simulink model "Airship_nonlinear_dynamics_simulink"  (R2024b)
settings: Solver=ode15s  StartTime=0.0  StopTime=1000  FixedStep=0.01  MaxStep=0.01  RelTol=1e-5  AbsTol=1e-8
InitFcn:
  | Init
values from neighbouring files (symbols this model uses):
  c = 0.465    [Init.m]    (also in Nonlinear_dynamics.m = 7; init_Skyship.m = 7)
  cf = 0.1395    [Init.m]    (also in Nonlinear_dynamics.m = 3; init_Skyship.m = 3)
  CL_alpha = 5.7    [Init.m]    (also in Nonlinear_dynamics.m; init_Skyship.m)
  D = 1.6    [Init.m]    (also in Nonlinear_dynamics.m = 14; init_Skyship.m = 14)
  delta = deg2rad(10)    [Nonlinear_dynamics.m]    (also in init_Skyship.m = -15)
  delta_e = 0    [Init.m]
  delta_r = 0    [Init.m]
  etaTDF = 1    [Init.m]    (also in Nonlinear_dynamics.m = 0.6; init_Skyship.m = 0.6)
  etaTP = 0.6    [Init.m]    (also in Nonlinear_dynamics.m; init_Skyship.m)
  fProp1 = 0    [Init.m]
  fProp2 = 0    [Init.m]
  fProp_max = 20    [Init.m]
  fTDF = 4000    [Nonlinear_dynamics.m]    (also in init_Skyship.m = 0)
  fTTP = 0    [Init.m]    (also in Nonlinear_dynamics.m = 2000; init_Skyship.m)
  FVN = [5, 5, 5]    [Init.m]    (also in Nonlinear_dynamics.m = 0; init_Skyship.m = 10)
  g = 9.81    [Init.m]    (also in Nonlinear_dynamics.m; init_Skyship.m)
  I33 = eye(3)    [Init.m]    (also in Nonlinear_dynamics.m; init_Skyship.m)
  Ixx = 1.7972    [Init.m]    (also in Nonlinear_dynamics.m = 200658; init_Skyship.m = 200658)
  Ixy = 0    [Init.m]    (also in Nonlinear_dynamics.m; init_Skyship.m)
  Ixz = 0    [Init.m]    (also in Nonlinear_dynamics.m; init_Skyship.m)
  Iyy = 4.9584    [Init.m]    (also in Nonlinear_dynamics.m = 850900; init_Skyship.m = 850900)
  Iyz = 0    [Init.m]    (also in Nonlinear_dynamics.m; init_Skyship.m)
  Izz = 7.9854    [Init.m]    (also in Nonlinear_dynamics.m = 649699; init_Skyship.m = 649699)
  k1 = keta(1)    [Init.m]    (also in Nonlinear_dynamics.m; init_Skyship.m = 0.08; ketaparameters.m = 0)
  k2 = keta(2)    [Init.m]    (also in Nonlinear_dynamics.m; init_Skyship.m = 0.89; ketaparameters.m = 0)
  k_dash = keta(3)    [Init.m]    (also in Nonlinear_dynamics.m; init_Skyship.m = 0.5; ketaparameters.m = 0)
  L = 4.7    [Init.m]    (also in Nonlinear_dynamics.m = zeros(1,4); init_Skyship.m = 52)
  m = 7.31    [Init.m]    (also in Nonlinear_dynamics.m = 5942; init_Skyship.m = 5942; velocity_tf_script.m; velocity_tf_script_v2.m)
  MAF = zeros(6,6)    [Init.m]    (also in Nonlinear_dynamics.m; init_Skyship.m)
  MVN = [0.2, 10, 5]    [Init.m]    (also in Nonlinear_dynamics.m = 0; init_Skyship.m = 0.001)
  p0 = 0    [Init.m]    (also in init_Skyship.m)
  phi0 = 0    [Init.m]    (also in init_Skyship.m)
  Prop1_alpha = 0    [Init.m]
  Prop2_alpha = 0    [Init.m]
  psi0 = 0    [Init.m]    (also in init_Skyship.m)
  q0 = 0    [Init.m]    (also in init_Skyship.m)
  r0 = 0    [Init.m]    (also in init_Skyship.m)
  rGxm = [XG-XB 0 ZG-ZB]'    [Init.m]    (also in Nonlinear_dynamics.m; init_Skyship.m)
  rho_0 = 1.225    [Init.m]    (also in Nonlinear_dynamics.m; init_Skyship.m)
  rho_he = 0.175    [Init.m]
  rTDF1 = [0 0.5 0]'    [Init.m]    (also in Nonlinear_dynamics.m = [3.5 7.87 21]'; init_Skyship.m = [3.5 7.87 21]')
  rTDF2 = [0 -0.5 0]'    [Init.m]    (also in Nonlinear_dynamics.m = [3.5 -7.87 21]'; init_Skyship.m = [3.5 -7.87 21]')
  rTTP = [0 0 0]'    [Init.m]    (also in Nonlinear_dynamics.m = [0 0 20.1]'; init_Skyship.m = [0 0 20.1]')
  Sf = 0.18135    [Init.m]    (also in Nonlinear_dynamics.m = 65; init_Skyship.m = 65)
  t_s = 0.005    [Init.m]
  theta0 = 1    [Init.m]    (also in init_Skyship.m = 0)
  u0 = 0.0    (= 0)    [Init.m]    (also in init_Skyship.m; velocity_tf_script.m = 4; velocity_tf_script_v2.m = 4)
  v0 = 0.0    (= 0)    [Init.m]    (also in init_Skyship.m)
  VB = 5.97    [Init.m]    (also in Nonlinear_dynamics.m = 5153; init_Skyship.m = 4911)
  w0 = 0.0    (= 0)    [Init.m]    (also in init_Skyship.m)
  xE0 = 0    [Init.m]    (also in init_Skyship.m)
  yE0 = 0    [Init.m]    (also in init_Skyship.m)
  zE0 = -h    (= -3.7495)    [Init.m]    (also in init_Skyship.m = -100)
undefined symbols (not defined in the file or in its folder): Sim3dSensor
libraries: slpidlib x13, simulink_extras x4, sim3dcameralib x1, sim3dlib x1, uavsim3dlib x1
(part 3 of 4)

== matlab function Airship_nonlinear_dynamics_simulink/nonlinear dynamics piecewise1/MATLAB Function6 ==
  data: phi input; g_cap output; theta input
function g_cap = fcn(phi, theta)
    g_cap = [-sin(theta), cos(theta)*sin(phi), cos(theta)*cos(phi)]';
end

== matlab function Airship_nonlinear_dynamics_simulink/nonlinear dynamics piecewise1/MATLAB Function7 ==
  data: rTDF1 input; tau_Th output; rTDF2 input; fProp1 input; fProp2 input; etaTDF input; rTTP input; fTTP input; etaTP input
function tau_Th = fcn(rTDF1, rTDF2, fProp1, fProp2, etaTDF, rTTP,  fTTP,  etaTP)
%% Airship thrust force and moments


FTDF1 = etaTDF * [fProp1 0 0 ]'; %Thrust force N
FTDF2 = etaTDF * [fProp2 0 0 ]';
FTDF = FTDF1+FTDF2;
MTDF1 = cross(rTDF1, FTDF1); %Moments N-m
MTDF2 = cross(rTDF2, FTDF2);
MTDF = MTDF1 + MTDF2;


FTTP = etaTP* [fTTP 0 0 ]';
MTTP = cross(rTTP, FTTP);

FT = FTTP + FTDF;
MT = MTTP + MTDF;
tau_Th = [FT; MT];
end

== matlab function Airship_nonlinear_dynamics_simulink/nonlinear dynamics piecewise1/V_dot out ==
  data: MAH input; V_dot output; MAF input; Mrigid input; tau_I input; tau_G input; tau_C input; tau_AS input; tau_A_dash input; tau_Th input; tau_V input
function V_dot = fcn(MAH, MAF, Mrigid,tau_I, tau_G, tau_C, tau_AS, tau_A_dash, tau_Th, tau_V)
%% Return
V_dot = zeros(6,1);
MA_rigid = (MAH+MAF);
%                                       +tau_Imp for gusts
V_dot = (MA_rigid + Mrigid) \ (tau_I + tau_G + tau_C + tau_AS + tau_A_dash + tau_Th + tau_V);
end

== matlab function Airship_nonlinear_dynamics_simulink/nonlinear dynamics piecewise1/tau_AS ==
  data: rho input; tau_AS output size=[6, 1]; g input; VB input; g_cap input; rho_he input
function tau_AS = fcn(rho, g, VB, g_cap, rho_he)
%% Aerostatic forces and moments

% first three are forces along x y z
% next three are moments along x y z 
rv = [0 0 0]'; %Since body frame is established at CV, the position ...
FAS = -(rho)*g*VB*g_cap; %Aerostatic forces N
%FAS = -((rho - rho_he) * g * VB) * g_cap;

tau_AS = [FAS; cross(rv,FAS)]; %Aerostatic forces and moments
end

== matlab function Airship_nonlinear_dynamics_simulink/Euler angle estimation2 ==
  data: phi input; EA_dot output; theta input; psi input; p input; q input; r input
function EA_dot = Euler_angle_estimation(phi, theta, psi,p, q, r)


E_dot = [1, sin(phi)* tan(theta) , cos(phi)*tan(theta);
         0, cos(phi) , -sin(phi);
         0, sin(phi)/cos(theta), cos(phi)/cos(theta)];

body_rates = [p; q; r];

EA_dot = transpose(E_dot*body_rates);

end

== matlab function Airship_nonlinear_dynamics_simulink/nonlinear dynamics piecewise1/tau_A_dash ==
  data: MA_rigid input; tau_A_dash output size=[6, 1]; omg input; V input
function tau_A_dash = fcn(MA_rigid, omg, V)
%% Aerodynamic forces and moments
% symmetric added mass axis
% Aerodynamic forces N and moments N-m

% Extract components from the symmetric added mass axis
M11 = MA_rigid(1:3, 1:3);
M12 = MA_rigid(1:3, 4:6);
M21 = MA_rigid(4:6, 1:3);
M22 = MA_rigid(4:6, 4:6);

% Calc aero forces and moments
forces_due_to_rotation = cross(omg, (M11 * V + M12 * omg));
moments_due_to_translation = cross(V, (M11 * V + M12 * omg));
moments_due_to_rotation = cross(omg, (M21 * V + M22 * omg));

% --- Pitch rate damping (natural, from hull and fins) ---
% Set this value using data for your airship (e.g. Skyship-500: -1.2e6 N·m·s/rad)
Mq = -1.2e6; % [N·m·s/rad] (example value, replace with your own if needed)
Mp = -1.2e6; % [N·m·s/rad] (example value, replace with your own if needed)

p = omg(1);

q = omg(2);  % Pitch rate (rad/s)
M_pitch_damping = Mq * q; % Negative sign already in Mq
M_yaw_damping = Mp * p; % Negative sign already in Mq

% Add pitch damping to the moment vector [L; M; N]
moments_due_to_pitch_damping = [0; M_pitch_damping; 0];
moments_due_to_yaw_damping = [M_yaw_damping;0; 0];

% Combine into aero forces and moments (sign change - to +)
tau_A_dash = [forces_due_to_rotation;
              moments_due_to_translation + moments_due_to_rotation + moments_due_to_pitch_damping+moments_due_to_yaw_damping];
end

== matlab function Airship_nonlinear_dynamics_simulink/nonlinear dynamics piecewise1/tau_C ==
  data: u input; tau_C output size=[6, 1]; v input; w input; delta_e input; delta_r input; rho input; Sf input; c input; cf input; CL_alpha input; L_hull input

function tau_C = fcn(u, v, w, delta_e, delta_r,rho, Sf, c, cf, CL_alpha, L_hull)
V_bar  = sqrt(u^2 + v^2 + w^2); % TAS m/s
S_FE   = Sf;                    % reference surface area m^2
delta_e_rad = deg2rad(delta_e);
delta_r_rad = deg2rad(delta_r);
q = 0.5 * rho * V_bar^2;
 
 %theoretical effectiveness factor tau
 theta_f = acos(2*cf/c -1);
 tau = 1- (theta_f - sin(theta_f)) /pi;
 
 %correction factor eta_d
 eta_d = 0.8; %simplified fucntion
 %3D effectiveness value
 k3D = 1.2; %example value
 %calc DeltaCL
 
 DeltaCL_elev = CL_alpha *tau * eta_d * k3D * delta_e_rad;
 DeltaCL_rud = CL_alpha *tau * eta_d * k3D * delta_r_rad;
 DeltaCD_elev = 1.7* (cf/c)^1.38 * (Sf / S_FE) * sin(delta_e_rad)^2;
 DeltaCD_rud = 1.7* (cf/c)^1.38 * (Sf / S_FE) * sin(delta_r_rad)^2; 
   %{
 %Moment calcs for each fin
 numerator = -2*sin(theta_f) - sin(2*theta_f);
 denominator = 8 * (pi - theta_f + sin(theta_f));

 ratio = numerator/denominator;

 DeltaCM1_4_elev = ratio*DeltaCL_elev;
 DeltaCM1_4_rud = ratio*DeltaCL_rud;

 %Deflection angels degrees
 theta = [90, 270, 0, 180];
  %}
 %initialize force and moment arrays
 
 Fx = zeros(1,4); %logitudinal forces
 Fy = zeros(1,4); %lateral forces
 Fz = zeros(1,4); %vertical forces
 
 L = zeros(1,4); %rolling moment
 M = zeros(1,4); %pitching moment
 N = zeros(1,4); %yawing moment
 
 %calc forces and moements for each fin
 
 for i = 1:2
 
     %calc forces
     Fx(i) = -q *Sf*DeltaCD_elev;
     Fy(i) = 0;
     Fz(i) = q*Sf*(DeltaCL_elev);
 
     L(i) = 0;
     M(i) = Fz(i)*0.5*L_hull; %assume moment arm is haf of the hull length
     N(i) = 0;
 end
 for i = 3:4
     %calc forces
     Fx(i) = -q *Sf*DeltaCD_rud;
     Fy(i) = -q *Sf*(DeltaCL_rud);
     Fz(i) = 0;
 
     L(i) = 0;
     M(i) = 0;
     N(i) = Fy(i)*0.5*L_hull; %assume moment arm is haf of the hull length
 end

 % Totals
 TotalFx = sum(Fx(:));
 TotalFy = sum(Fy(:));
 TotalFz = sum(Fz(:));

 TotalL = sum(L(:));
 TotalM = sum(M(:));
 TotalN = sum(N(:));
 tau_C = [TotalFx TotalFy TotalFz TotalL TotalM TotalN]';


end
%{
function tau_C = fcn(u, v, w, delta, rho, Sf, c, cf, CL_alpha)
% fcn computes the forces and moments exerted by the elevator.
%
% Syntax:
%   tau_C = fcn(u, v, w, delta, rho, Sf, c, cf, CL_alpha)
%
% Inputs:
%   u, v, w   - Velocities in the body axes (m/s)
%   delta     - Elevator deflection (in degrees)
%   rho       - Air density (kg/m^3)
%   Sf        - Fin (or elevator) surface area (m^2)
%   c         - Chord length of the fin (m)
%   cf        - Chord length of the flap (m)
%   CL_alpha  - Lift curve slope (per radian)
%
% Outputs:
%   tau_C     - 6x1 column vector with total force and moment components:
%               [TotalFx; TotalFy; TotalFz; TotalL; TotalM; TotalN]
%
% The function computes the force generated by the elevator using a
% simplified aerodynamic model. Later, rudder contributions can be added.
%

% -------------------------------------------------
% Constants and preliminary calculations
% -------------------------------------------------
V_bar  = sqrt(u^2 + v^2 + w^2);        % true airspeed in m/s
S_FE   = Sf;                           % reference surface area m^2
delta_rad = deg2rad(delta);            % convert deflection to radians

% Deflection angles (degrees) for all 4 fins (2 elevator and 2 rudder)
theta = [45, 135, 225, 315];

% -------------------------------------------------
% Initialize force and moment arrays
% -------------------------------------------------
% Force components (assumed to be calculated for each fin/elevator)
Fx = zeros(size(theta));  % X forces (e.g., drag)
Fy = zeros(size(theta));  % Y forces (lateral - zero in symmetric case)
Fz = zeros(size(theta));  % Z forces (lift)

% Moment components for each fin/elevator
L = zeros(size(theta));  % Rolling moment about x-axis
M = zeros(size(theta));  % Pitching moment about y-axis
N = zeros(size(theta));  % Yawing moment about z-axis

% -------------------------------------------------
% Aerodynamic force calculations
% -------------------------------------------------
% Calculate dynamic pressure
q = 0.5 * rho * V_bar^2;

% Elevator lift (simplified linear model)
% Using the relation: Lift = q * S_FE * CL_alpha * delta_rad
Lift = q * S_FE * CL_alpha * delta_rad;

% For this example, we assume that all 4 fins (or elevator surfaces)
% produce identical contributions. More nuanced models would separately
% handle the contributions from elevator vs. rudder.
%
% Here we distribute the forces and moments for each surface.
for i = 1:length(theta)
    % Forces:
    % - Fx: a small fraction (e.g., 10%) of the lift is assumed to be
    %       converted to a drag force along the x-axis.
    % - Fy: no lateral force is assumed (symmetry).
    % - Fz: the full lift is assumed to act in the vertical direction.
    Fx(i) = 0.1 * Lift;
    Fy(i) = 0;
    Fz(i) = Lift;
    
    % Moments (using chord as approximate lever arms):
    % - Rolling moment (L): assumed to be 0.5 * Lift * c
    % - Pitching moment (M): assumed to be Lift * c
    % - Yawing moment (N): assumed to be 0.5 * Lift * cf
    L(i) = 0.5 * Lift * c;
    M(i) = Lift * c;
    N(i) = 0.5 * Lift * cf;
end

% -------------------------------------------------
% Consolidate the total forces and moments
% -------------------------------------------------
TotalFx = sum(Fx(:));
TotalFy = sum(Fy(:));
TotalFz = sum(Fz(:));

TotalL  = sum(L(:));
TotalM  = sum(M(:));
TotalN  = sum(N(:));

% Output: Force and moment vector as a column vector
tau_C = [TotalFx; TotalFy; TotalFz; TotalL; TotalM; TotalN];

end
%}
%{ 
%% Control forces and moments
% Constants
 V_bar  = sqrt(v^2 + u^2 + w^2) ; %true airspeed in m/s
 S_FE = Sf; %reference surface area m^2
 delta_rad = deg2rad(delta);
 
 %theoretical effectiveness factor tau
 theta_f = acos(2*cf/c -1);
 tau = 1- (theta_f - sin(theta_f)) /pi;
 
 %correction factor eta_d
 eta_d = 0.8; %simplified fucntion
 %3D effectiveness value
 k3D = 1.2; %example value
 %calc DeltaCL
 
 DeltaCL = CL_alpha *tau * eta_d * k3D * delta_rad;
 
 DeltaCD = 1.7* (cf/c)^1.38 * (Sf / S_FE) * sin(delta_rad)^2;
 
 %Moment calcs for each fin
 numerator = -2*sin(theta_f) - sin(2*theta_f);
 denominator = 8 * (pi - theta_f + sin(theta_f));
 
 ratio = numerator/denominator;
 
 DeltaCM1_4 = ratio*DeltaCL;
 
 %Deflection angels degrees
 theta = [45, 135, 225, 315];
 
 %initialize force and moment arrays
 
 Fx = zeros(1,4);
 Fy = zeros(1,4);
 Fz = zeros(1,4);
 
 L = zeros(1,4);
 M = zeros(1,4);
 N = zeros(1,4);
 
 %calc forces and moements for each fin
 
 for i = 1:4
     %conv theta to radians
     theta_rad = deg2rad(theta(i));
 
     %calc forces
     Fx(i) = -0.5 * rho * V_bar^2 *Sf*DeltaCD;
     Fy(i) = 0.5*rho*V_bar^2*Sf*(DeltaCL *sin(theta_rad)+ DeltaCD * cos(theta_rad));
     Fz(i) = -0.5 * rho * V_bar^2 *Sf*(DeltaCL *cos(theta_rad)- DeltaCD * sin(theta_rad));
 
     L(i) = Fz(i); %Assume y_i = 1 for simplicity
     M(i) = 0.5*rho*V_bar^2*Sf*c*DeltaCM1_4;
     N(i) = Fy(i); %Assume x_i = 1 for simplicity 
 end
 % Totals
 TotalFx = sum(Fx(:));
 TotalFy = sum(Fy(:));
 TotalFz = sum(Fz(:));

 TotalL = sum(L(:));
 TotalM = sum(M(:));
 TotalN = sum(N(:));
 tau_C = [TotalFx TotalFy TotalFz TotalL TotalM TotalN]';


end
%For natural response 
%tau_C = [0 0 0 0 0 0]';
%}

== matlab function Airship_nonlinear_dynamics_simulink/nonlinear dynamics piecewise1/tau_G ==
  data: rho input; tau_G output size=[6, 1]; m input; g input; VB input; rGx input; g_cap input
function tau_G = fcn(rho, m, g, VB, rGx, g_cap)
%% Gravitational forces and moments
w = m*g;

FG = w*g_cap; % Weight component in body frame (N)
tau_G = [FG; rGx*FG];
end

== matlab function Airship_nonlinear_dynamics_simulink/nonlinear dynamics piecewise1/tau_I ==
  data: J input; tau_I output size=[6, 1]; rGx input; p input; q input; r input; V input; omg input; m input
function tau_I = fcn(J, rGx, p, q, r, V, omg,m)
%% Inertial forces (N) and moments (N-m)
omgx = [0 -omg(3) omg(2) ; omg(3) 0 -omg(1) ; -omg(2) omg(1) 0];

tau_I = [-m*omgx*V + m*omgx*rGx*omg ; -m*rGx*omgx*V - omgx*J*omg];
end

== matlab function Airship_nonlinear_dynamics_simulink/Euler angle estimation4 ==
  data: phi input; EA_dot output; theta input; psi input; p input; q input; r input
function EA_dot = Euler_angle_estimation(phi, theta, psi,p, q, r)


E_dot = [1, sin(phi)* tan(theta) , cos(phi)*tan(theta);
         0, cos(phi) , -sin(phi);
         0, sin(phi)/cos(theta), cos(phi)/cos(theta)];

body_rates = [p; q; r];

EA_dot = transpose(E_dot*body_rates);

end

== matlab function Airship_nonlinear_dynamics_simulink/Position wrt earth4 ==
  data: u input; XYZ_dot output; v input; w input; phi input; theta input; psi input
function XYZ_dot = position_wrt_Earth(u,v,w,phi,theta,psi)


R_be = [cos(theta)*cos(psi) , sin(theta)*sin(phi)*cos(psi) - cos(theta)*sin(psi), cos(phi)*cos(psi)*sin(theta)+ sin(phi)*sin(psi); ...
    cos(theta)*sin(psi), sin(phi)*sin(theta)*sin(psi) + cos(phi)*cos(psi), cos(phi)*sin(theta)*sin(psi) - sin(phi)*cos(psi); ...
    -sin(theta) , sin(phi)*cos(theta) , cos(phi)*cos(theta)];

body_velocity = [u; v; w];
XYZ_dot = transpose(R_be*body_velocity);
end

== matlab function Airship_nonlinear_dynamics_simulink/nonlinear dynamics piecewise2/MATLAB Function ==
  data: u input; V_dot output size=[6, 1]; v input; w input; p input; q input; r input; phi input; theta input; psi input; Z input; MAF input; m input; I33 input; rGxm input; Ixx input; Iyy input; Izz input; Ixy input; Ixz input; Iyz input; g input; L input; D input; k1 input; k2 input; k_dash input; VB input; delta input; rTDF1 input; rTDF2 input; fTDF input; etaTDF input; rTTP input; fTTP input; etaTP input
function V_dot = fcn(u, v, w, p, q, r, phi, theta, psi, Z, MAF, m, I33, rGxm, Ixx, Iyy, Izz, Ixy, Ixz, Iyz, g, L, D, k1, k2, k_dash, VB, delta, rTDF1, rTDF2, fTDF, etaTDF, rTTP,  fTTP,  etaTP)
rGx = [0 -rGxm(3) rGxm(2) ; rGxm(3) 0 -rGxm(1) ; -rGxm(2) rGxm(1) 0];
J = [ Ixx, Ixy, Ixz ; Ixy, Iyy, Iyz ; Ixz, Iyz, Izz];
Mrigid = [m*I33, -m*rGx; m*rGx,  J];
g_cap = [-sin(theta), cos(theta)*sin(phi), cos(theta)*cos(phi)]';
V = [u v w]';
omg = [p q r]';
altitude = -Z;
rho_0 = 1.225; %Density at sea level in kg/m3
H = 8400; %Scale height in meters;
%alitude range
%altitude = -airship(12); %linspace(0,12000, 500); %Altitude from 0 to 12000 m
density = rho_0 *exp(-altitude / H );
rho = density;

%% Estimation of added mass matrix
% MAH - added mass of airship hull
B = VB*rho*g; %Bouyancy force
m_dash = B/g;
%I_dash = sum(m_dash * (L.^2 + D^2) / 20); 
I_dash = (m_dash * (L.^2 + D^2) / 20); 
mH11 = k1*m_dash;
mH22 = k2*m_dash;
mH33 = mH22;
mH44 = 0;
mH55 = k_dash*I_dash;
mH66 = mH55;
mH = [mH11, mH22, mH33, mH44, mH55, mH66];
MAH = diag(mH); %6x6 diagonal matrix

MA_rigid = (MAH+MAF);

%% Inertial forces (N) and moments (N-m)
omgx = [0 -omg(3) omg(2) ; omg(3) 0 -omg(1) ; -omg(2) omg(1) 0];
tau_I = [-m*omgx*V + m*omgx*rGx*omg ; -m*rGx*omgx*V - omgx*J*omg];

%% Gravitational forces and moments
w = m*g;
B = VB*rho*g;
FG = w*g_cap; % Weight component in body frame (N)
tau_G = [FG; rGx*FG];

%% Control forces and moments
% Constants

 V_bar  = sqrt(v^2 + u^2 + w^2) ; %true airspeed in m/s
 Sf = 65; % Surface area of the fin m^2
 c= 7 ; % Chord length of the fin
 cf = 3; %Flap chord
 
 S_FE = 65; %reference surface area m^2
 %
 delta_rad = deg2rad(delta);
 %lift curve slope
 CL_alpha = 5.7; %Change as needed
 
 %theoretical effectiveness factor tau
 theta_f = acos(2*cf/c -1);
 tau = 1- (theta_f - sin(theta_f)) /pi;
 
 %correction factor eta_d
 eta_d = 0.8; %simplified fucntion
 %3D effectiveness value
 k3D = 1.2; %example value
 %calc DeltaCL
 
 DeltaCL = CL_alpha *tau * eta_d * k3D * delta_rad;
 
 DeltaCD = 1.7* (cf/c)^1.38 * (Sf / S_FE) * sin(delta_rad)^2;
 
 %Moment calcs for each fin
 numerator = -2*sin(theta_f) - sin(2*theta_f);
 denominator = 8 * (pi - theta_f + sin(theta_f));
 
 ratio = numerator/denominator;
 
 DeltaCM1_4 = ratio*DeltaCL;
 
 %Deflection anges degrees
 theta = [45, 135, 225, 315];
 
 %initialize force and moment arrays
 
 Fx = zeros(1,4);
 Fy = zeros(1,4);
 Fz = zeros(1,4);
 
 L = zeros(1,4);
 M = zeros(1,4);
 N = zeros(1,4);
 
 %calc forces and moements for each fin
 
 for i = 1:4
     %conv theta to radians
     theta_rad = deg2rad(theta(i));
 
     %calc forces
     Fx(i) = -0.5 * rho * V_bar^2 *Sf*DeltaCD;
     Fy(i) = 0.5*rho*V_bar^2*Sf*(DeltaCL *sin(theta_rad)+ DeltaCD * cos(theta_rad));
     Fz(i) = -0.5 * rho * V_bar^2 *Sf*(DeltaCL *cos(theta_rad)- DeltaCD * sin(theta_rad));
 
     L(i) = Fz(i); %Assume y_i = 1 for simplicity
     M(i) = 0.5*rho*V_bar^2*Sf*c*DeltaCM1_4;
     N(i) = Fy(i); %Assume x_i = 1 for simplicity 
 end
 % Totals
 TotalFx = sum(Fx(:));
 TotalFy = sum(Fy(:));
 TotalFz = sum(Fz(:));

 TotalL = sum(L(:));
 TotalM = sum(M(:));
 TotalN = sum(N(:));
 tau_C = [TotalFx TotalFy TotalFz TotalL TotalM TotalN]';
%For natural response 
%tau_C = [0 0 0 0 0 0]';

%% Aerostatic forces and moments

% first three are forces along x y z
% next three are moments along x y z 
rv = [0 0 0]'; %Since body frame is established at CV, the position ...
FAS = -rho*g*VB*g_cap; %Aerostatic forces N
tau_AS = [FAS; cross(rv,FAS)]; %Aerostatic forces and moments

%% Aerodynamic forces and moments
% symmetric added mass axis
% Aerodynamic forces N and moments N-m

%extract components from the syymetric added mass axis
M11 = MA_rigid(1:3, 1:3);
M12 = MA_rigid(1:3, 4:6);
M21 = MA_rigid(4:6, 1:3);
M22 = MA_rigid(4:6, 4:6);

% Calc aero forces and moments

forces_due_to_rotation = cross(omg, (M11 * V + M12 *omg));
moments_due_to_translation = cross(V, (M11*V+M12*omg));
moments_due_to_rotation = cross (omg, (M21*V + M22*omg));

tau_A_dash = zeros(6,1);
%combine into aero forces and moments (sign change - to +)
tau_A_dash = [forces_due_to_rotation; moments_due_to_translation+moments_due_to_rotation];

%% Airship thrust force and moments


FTDF1 = etaTDF * [fTDF 0 0 ]'; %Thrust force N
FTDF2 = etaTDF * [fTDF 0 0 ]';
FTDF = FTDF1+FTDF2;
MTDF1 = cross(rTDF1, FTDF1); %Moments N-m
MTDF2 = cross(rTDF2, FTDF2);
MTDF = MTDF1 + MTDF2;


FTTP = etaTP* [fTTP 0 0 ]';
MTTP = cross(rTTP, FTTP);

FT = FTTP + FTDF;
MT = MTTP + MTDF;
tau_Th = [FT; MT];

%% Viscous forces
FVN = 0; %Viscous force
MVN = 0; %Viscous Moment

if v == 0 && w == 0
    FV = [0 0 0]';
    MV = [0 0 0]';
else
    FV = FVN*[0 (-v/sqrt(v^2 + w^2)) (-w/sqrt(v^2 +w^2)) ]';
    MV = MVN*[0 (w/sqrt(v^2 + w^2)) (-v/sqrt(v^2 +w^2)) ]';
end
tau_V = [FV; MV];

%tau_V = [0 0 0 0 0 0]'; %if slow speed


%% Return
V_dot = zeros(6,1);
MA_rigid = (MAH+MAF);


%                                       +tau_Imp for gusts
V_dot = (MA_rigid + Mrigid) \ (tau_I + tau_G + tau_C + tau_AS + tau_A_dash + tau_Th + tau_V);

== matlab function Airship_nonlinear_dynamics_simulink/nonlinear dynamics piecewise/tau_I ==
  data: J input; tau_I output size=[6, 1]; rGx input; p input; q input; r input; V input; omg input
function tau_I = fcn(J, rGx, p, q, r, V, omg)
%% Inertial forces (N) and moments (N-m)
omgx = [0 -omg(3) omg(2) ; omg(3) 0 -omg(1) ; -omg(2) omg(1) 0];

tau_I = [-m*omgx*V + m*omgx*rGx*omg ; -m*rGx*omgx*V - omgx*J*omg];

== matlab function Airship_nonlinear_dynamics_simulink/Airship_model/Euler angle estimation5 ==
  data: phi input; EA_dot output; theta input; psi input; p input; q input; r input
function EA_dot = Euler_angle_estimation(phi, theta, psi,p, q, r)


E_dot = [1, sin(phi)* tan(theta) , cos(phi)*tan(theta);
         0, cos(phi) , -sin(phi);
         0, sin(phi)/cos(theta), cos(phi)/cos(theta)];

body_rates = [p; q; r];

EA_dot = transpose(E_dot*body_rates);

end

== matlab function Airship_nonlinear_dynamics_simulink/Airship_model/Position wrt earth5 ==
  data: u input; XYZ_dot output; v input; w input; phi input; theta input; psi input
function XYZ_dot = position_wrt_Earth(u,v,w,phi,theta,psi)


R_be = [cos(theta)*cos(psi) , sin(theta)*sin(phi)*cos(psi) - cos(theta)*sin(psi), cos(phi)*cos(psi)*sin(theta)+ sin(phi)*sin(psi); ...
    cos(theta)*sin(psi), sin(phi)*sin(theta)*sin(psi) + cos(phi)*cos(psi), cos(phi)*sin(theta)*sin(psi) - sin(phi)*cos(psi); ...
    -sin(theta) , sin(phi)*cos(theta) , cos(phi)*cos(theta)];

body_velocity = [u; v; w];
XYZ_dot = transpose(R_be*body_velocity);
end

== matlab function Airship_nonlinear_dynamics_simulink/Airship_model/nonlinear dynamics piecewise3/MAH ==
  data: MAH output; g input; L input; D input; k1 input; k2 input; k_dash input; VB input; rho input
function MAH = fcn(g, L, D, k1, k2, k_dash, VB, rho)
%% Estimation of added mass matrix
% MAH - added mass of airship hull
B = VB*rho*g; %Bouyancy force
m_dash = B/g;
%I_dash = sum(m_dash * (L.^2 + D^2) / 20); 
I_dash = (m_dash * (L.^2 + D^2) / 20); 

mH11 = k1*m_dash;
mH22 = k2*m_dash;
mH33 = mH22;
mH44 = 0;
mH55 = k_dash*I_dash;
mH66 = mH55;
mH = [mH11, mH22, mH33, mH44, mH55, mH66];

MAH = diag(mH); %6x6 diagonal matrix
end

== matlab function Airship_nonlinear_dynamics_simulink/Airship_model/nonlinear dynamics piecewise3/MATLAB Function10 ==
  data: u input; V output; v input; w input
function V = fcn(u, v, w)
V = [u v w]';
end

== matlab function Airship_nonlinear_dynamics_simulink/Airship_model/nonlinear dynamics piecewise3/MATLAB Function11 ==
  data: V input; r input; q input; tau_V output size=[6,1]; MVN input; FVN input
 function tau_V = fcn(V, r,q, MVN, FVN)
 u= V(1); 
 v = V(2);
 w= V(3);

 if v == 0 && w == 0
     FV = [0 0 0]';
     MV = [0 0 0]';
 else
     FV = FVN.*[-u (-v) (-w) ]';
     %FV = FVN*[0 (-v/sqrt(v^2 + w^2)) (-w/sqrt(v^2 +w^2)) ]';
     %MV = MVN*[0 (w/sqrt(v^2 + w^2)) (-v/sqrt(v^2 +w^2)) ]';
    MV = MVN.*[0 (w) (-v) ]'; %make first element function of p if roll oscilations persists

 end
 MV(3) = MV(3) - MVN(3) * r; 
 MV(2) = MV(2) - MVN(2) * q;
 tau_V = [FV; MV];
 %tau_V = [0 0 0 0 0 0]'; %if slow speed
 
 end

== matlab function Airship_nonlinear_dynamics_simulink/Airship_model/nonlinear dynamics piecewise3/MATLAB Function14 ==
  data: altitude input; rho output; rho_0 input
function rho = fcn(altitude, rho_0)
    % Constants
    T0 = 288.15;     % K
    L = 0.0065;      % K/m
    g = 9.80665;     % m/s^2
    R = 287.05;      % J/kg.K
%altitude = max(0, altitude);  % keep ≥ 0, but not forcefully clipped
    term = 1 - (L * altitude) / T0;
%rho= rho_0;
    if term <= 0
        rho = 0;
    else
       rho = rho_0 * term^(g / (R * L));
    end
end

== matlab function Airship_nonlinear_dynamics_simulink/Airship_model/nonlinear dynamics piecewise3/MATLAB Function15 ==
  data: p input; omg output; q input; r input
function omg = fcn(p, q, r)
omg = [p q r]';
end

== matlab function Airship_nonlinear_dynamics_simulink/Airship_model/nonlinear dynamics piecewise3/MATLAB Function2 ==
  data: rGxm input; rGx output
function rGx = fcn(rGxm)
rGx = [0 -rGxm(3) rGxm(2) ; rGxm(3) 0 -rGxm(1) ; -rGxm(2) rGxm(1) 0];

end

== matlab function Airship_nonlinear_dynamics_simulink/Airship_model/nonlinear dynamics piecewise3/MATLAB Function3 ==
  data: Ixx input; J output; Iyy input; Izz input; Ixy input; Ixz input; Iyz input
function J = fcn(Ixx, Iyy, Izz, Ixy, Ixz, Iyz)
J = [ Ixx, Ixy, Ixz ; Ixy, Iyy, Iyz ; Ixz, Iyz, Izz];
end

== matlab function Airship_nonlinear_dynamics_simulink/Airship_model/nonlinear dynamics piecewise3/MATLAB Function4 ==
  data: m input; Mrigid output; I33 input; rGx input; J input
function Mrigid = fcn(m, I33, rGx, J)
Mrigid = [m*I33, -m*rGx; m*rGx,  J];

end

== matlab function Airship_nonlinear_dynamics_simulink/Airship_model/nonlinear dynamics piecewise3/MATLAB Function6 ==
  data: phi input; g_cap output; theta input
function g_cap = fcn(phi, theta)
    g_cap = [-sin(theta), cos(theta)*sin(phi), cos(theta)*cos(phi)]';
end

== matlab function Airship_nonlinear_dynamics_simulink/Airship_model/nonlinear dynamics piecewise3/MATLAB Function7 ==
  data: rTDF1 input; tau_Th output; rTDF2 input; fProp1 input; fProp2 input; etaTDF input; Prop1_alpha input; Prop2_alpha input
function tau_Th = fcn(rTDF1, rTDF2, fProp1, fProp2, etaTDF, Prop1_alpha, Prop2_alpha)
%% Airship thrust force and moments


FTDF1 = etaTDF * [fProp1*cos(Prop1_alpha) 0 -fProp1*sin(Prop1_alpha)]'; %Thrust force N
FTDF2 = etaTDF * [fProp2*cos(Prop2_alpha) 0 -fProp2*sin(Prop2_alpha)]';
FTDF = FTDF1+FTDF2;
MTDF1 = cross(rTDF1, FTDF1); %Moments N-m
MTDF2 = cross(rTDF2, FTDF2);
MTDF = MTDF1 + MTDF2;

tau_Th = [FTDF; MTDF];
end

== matlab function Airship_nonlinear_dynamics_simulink/Airship_model/nonlinear dynamics piecewise3/V_dot out ==
  data: MAH input; V_dot output; MAF input; Mrigid input; tau_I input; tau_G input; tau_C input; tau_AS input; tau_A_dash input; tau_Th input; tau_V input
function V_dot = fcn(MAH, MAF, Mrigid,tau_I, tau_G, tau_C, tau_AS, tau_A_dash, tau_Th, tau_V)
%% Return
V_dot = zeros(6,1);
MA_rigid = (MAH+MAF);
%                                       +tau_Imp for gusts
V_dot = (MA_rigid + Mrigid) \ (tau_I + tau_G + tau_C + tau_AS + tau_A_dash + tau_Th + tau_V);
end

== matlab function Airship_nonlinear_dynamics_simulink/Position wrt earth2 ==
  data: u input; XYZ_dot output; v input; w input; phi input; theta input; psi input
function XYZ_dot = position_wrt_Earth(u,v,w,phi,theta,psi)


R_be = [cos(theta)*cos(psi) , sin(theta)*sin(phi)*cos(psi) - cos(theta)*sin(psi), cos(phi)*cos(psi)*sin(theta)+ sin(phi)*sin(psi); ...
    cos(theta)*sin(psi), sin(phi)*sin(theta)*sin(psi) + cos(phi)*cos(psi), cos(phi)*sin(theta)*sin(psi) - sin(phi)*cos(psi); ...
    -sin(theta) , sin(phi)*cos(theta) , cos(phi)*cos(theta)];

body_velocity = [u; v; w];
XYZ_dot = transpose(R_be*body_velocity);
end

== matlab function Airship_nonlinear_dynamics_simulink/Airship_model/nonlinear dynamics piecewise3/tau_AS ==
  data: rho input; tau_AS output size=[6, 1]; g input; VB input; g_cap input; rho_he input
function tau_AS = fcn(rho, g, VB, g_cap, rho_he)
%% Aerostatic forces and moments

% first three are forces along x y z
% next three are moments along x y z 
rv = [0 0 0]'; %Since body frame is established at CV, the position vector is 0
FAS = -(rho)*g*VB*g_cap; %Aerostatic forces N
%FAS = -((rho - rho_he) * g * VB) * g_cap;

tau_AS = [FAS; cross(rv,FAS)]; %Aerostatic forces and moments
end

== matlab function Airship_nonlinear_dynamics_simulink/Airship_model/nonlinear dynamics piecewise3/tau_A_dash ==
  data: MA_rigid input; tau_A_dash output size=[6, 1]; omg input; V input
function tau_A_dash = fcn(MA_rigid, omg, V)
%% Aerodynamic forces and moments
% symmetric added mass axis
% Aerodynamic forces N and moments N-m

% Extract components from the symmetric added mass axis
M11 = MA_rigid(1:3, 1:3);
M12 = MA_rigid(1:3, 4:6);
M21 = MA_rigid(4:6, 1:3);
M22 = MA_rigid(4:6, 4:6);

% Calc aero forces and moments
forces_due_to_rotation = cross(omg, (M11 * V + M12 * omg));
moments_due_to_translation = cross(V, (M11 * V + M12 * omg));
moments_due_to_rotation = cross(omg, (M21 * V + M22 * omg));

% --- Pitch rate damping (natural, from hull and fins) ---
% Set this value using data for your airship (e.g. Skyship-500: -1.2e6 N·m·s/rad)
Mq = -1.2e6; % [N·m·s/rad] (example value, replace with your own if needed)
Mp = -1.2e6; % [N·m·s/rad] (example value, replace with your own if needed)

p = omg(1);

q = omg(2);  % Pitch rate (rad/s)
M_pitch_damping = Mq * q; % Negative sign already in Mq
M_yaw_damping = Mp * p; % Negative sign already in Mq

% Add pitch damping to the moment vector [L; M; N]
moments_due_to_pitch_damping = [0; M_pitch_damping; 0];
moments_due_to_yaw_damping = [M_yaw_damping;0; 0];

% Combine into aero forces and moments (sign change - to +)
tau_A_dash = [forces_due_to_rotation;
              moments_due_to_translation + moments_due_to_rotation + moments_due_to_pitch_damping+moments_due_to_yaw_damping];
end

== matlab function Airship_nonlinear_dynamics_simulink/Airship_model/nonlinear dynamics piecewise3/tau_C ==
  data: u input; tau_C output size=[6, 1]; v input; w input; delta_e input; delta_r input; rho input; Sf input; c input; cf input; CL_alpha input; L_hull input

function tau_C = fcn(u, v, w, delta_e, delta_r,rho, Sf, c, cf, CL_alpha, L_hull)
V_bar  = sqrt(u^2 + v^2 + w^2); % TAS m/s
S_FE   = Sf;                    % reference surface area m^2
delta_e_rad = deg2rad(delta_e);
delta_r_rad = deg2rad(delta_r);
q = 0.5 * rho * V_bar^2;
 
 %theoretical effectiveness factor tau
 theta_f = acos(2*cf/c -1);
 tau = 1- (theta_f - sin(theta_f)) /pi;
 
 %correction factor eta_d
 eta_d = 0.8; %simplified fucntion
 %3D effectiveness value
 k3D = 1.2; %example value
 %calc DeltaCL
 
 DeltaCL_elev = CL_alpha *tau * eta_d * k3D * delta_e_rad;
 DeltaCL_rud = CL_alpha *tau * eta_d * k3D * delta_r_rad;
 DeltaCD_elev = 1.7* (cf/c)^1.38 * (Sf / S_FE) * sin(delta_e_rad)^2;
 DeltaCD_rud = 1.7* (cf/c)^1.38 * (Sf / S_FE) * sin(delta_r_rad)^2; 
   %{
 %Moment calcs for each fin
 numerator = -2*sin(theta_f) - sin(2*theta_f);
 denominator = 8 * (pi - theta_f + sin(theta_f));

 ratio = numerator/denominator;

 DeltaCM1_4_elev = ratio*DeltaCL_elev;
 DeltaCM1_4_rud = ratio*DeltaCL_rud;

 %Deflection angels degrees
 theta = [90, 270, 0, 180];
  %}
 %initialize force and moment arrays
 
 Fx = zeros(1,4); %logitudinal forces
 Fy = zeros(1,4); %lateral forces
 Fz = zeros(1,4); %vertical forces
 
 L = zeros(1,4); %rolling moment
 M = zeros(1,4); %pitching moment
 N = zeros(1,4); %yawing moment
 
 %calc forces and moements for each fin
 
 for i = 1:2
 
     %calc forces
     Fx(i) = -q *Sf*DeltaCD_elev;
     Fy(i) = 0;
     Fz(i) = -q*Sf*(DeltaCL_elev);
 
     L(i) = 0;
     M(i) = Fz(i)*0.5*L_hull; %assume moment arm is haf of the hull length
     N(i) = 0;
 end
 for i = 3:4
     %calc forces
     Fx(i) = -q *Sf*DeltaCD_rud;
     Fy(i) = q *Sf*(DeltaCL_rud);
     Fz(i) = 0;
 
     L(i) = 0;
     M(i) = 0;
     N(i) = Fy(i)*0.5*L_hull; %assume moment arm is haf of the hull length
 end

 % Totals
 TotalFx = sum(Fx(:));
 TotalFy = sum(Fy(:));
 TotalFz = sum(Fz(:));

 TotalL = sum(L(:));
 TotalM = sum(M(:));
 TotalN = sum(N(:));
 tau_C = [TotalFx TotalFy TotalFz TotalL TotalM TotalN]';


end
%{
function tau_C = fcn(u, v, w, delta, rho, Sf, c, cf, CL_alpha)
% fcn computes the forces and moments exerted by the elevator.
%
% Syntax:
%   tau_C = fcn(u, v, w, delta, rho, Sf, c, cf, CL_alpha)
%
% Inputs:
%   u, v, w   - Velocities in the body axes (m/s)
%   delta     - Elevator deflection (in degrees)
%   rho       - Air density (kg/m^3)
%   Sf        - Fin (or elevator) surface area (m^2)
%   c         - Chord length of the fin (m)
%   cf        - Chord length of the flap (m)
%   CL_alpha  - Lift curve slope (per radian)
%
% Outputs:
%   tau_C     - 6x1 column vector with total force and moment components:
%               [TotalFx; TotalFy; TotalFz; TotalL; TotalM; TotalN]
%
% The function computes the force generated by the elevator using a
% simplified aerodynamic model. Later, rudder contributions can be added.
%

% -------------------------------------------------
% Constants and preliminary calculations
% -------------------------------------------------
V_bar  = sqrt(u^2 + v^2 + w^2);        % true airspeed in m/s
S_FE   = Sf;                           % reference surface area m^2
delta_rad = deg2rad(delta);            % convert deflection to radians

% Deflection angles (degrees) for all 4 fins (2 elevator and 2 rudder)
theta = [45, 135, 225, 315];

% -------------------------------------------------
% Initialize force and moment arrays
% -------------------------------------------------
% Force components (assumed to be calculated for each fin/elevator)
Fx = zeros(size(theta));  % X forces (e.g., drag)
Fy = zeros(size(theta));  % Y forces (lateral - zero in symmetric case)
Fz = zeros(size(theta));  % Z forces (lift)

% Moment components for each fin/elevator
L = zeros(size(theta));  % Rolling moment about x-axis
M = zeros(size(theta));  % Pitching moment about y-axis
N = zeros(size(theta));  % Yawing moment about z-axis

% -------------------------------------------------
% Aerodynamic force calculations
% -------------------------------------------------
% Calculate dynamic pressure
q = 0.5 * rho * V_bar^2;

% Elevator lift (simplified linear model)
% Using the relation: Lift = q * S_FE * CL_alpha * delta_rad
Lift = q * S_FE * CL_alpha * delta_rad;

% For this example, we assume that all 4 fins (or elevator surfaces)
% produce identical contributions. More nuanced models would separately
% handle the contributions from elevator vs. rudder.
%
% Here we distribute the forces and moments for each surface.
for i = 1:length(theta)
    % Forces:
    % - Fx: a small fraction (e.g., 10%) of the lift is assumed to be
    %       converted to a drag force along the x-axis.
    % - Fy: no lateral force is assumed (symmetry).
    % - Fz: the full lift is assumed to act in the vertical direction.
    Fx(i) = 0.1 * Lift;
    Fy(i) = 0;
    Fz(i) = Lift;
    
    % Moments (using chord as approximate lever arms):
    % - Rolling moment (L): assumed to be 0.5 * Lift * c
    % - Pitching moment (M): assumed to be Lift * c
    % - Yawing moment (N): assumed to be 0.5 * Lift * cf
    L(i) = 0.5 * Lift * c;
    M(i) = Lift * c;
    N(i) = 0.5 * Lift * cf;
end

% -------------------------------------------------
% Consolidate the total forces and moments
% -------------------------------------------------
TotalFx = sum(Fx(:));
TotalFy = sum(Fy(:));
TotalFz = sum(Fz(:));

TotalL  = sum(L(:));
TotalM  = sum(M(:));
TotalN  = sum(N(:));

% Output: Force and moment vector as a column vector
tau_C = [TotalFx; TotalFy; TotalFz; TotalL; TotalM; TotalN];

end
%}
%{ 
%% Control forces and moments
% Constants
 V_bar  = sqrt(v^2 + u^2 + w^2) ; %true airspeed in m/s
 S_FE = Sf; %reference surface area m^2
 delta_rad = deg2rad(delta);
 
 %theoretical effectiveness factor tau
 theta_f = acos(2*cf/c -1);
 tau = 1- (theta_f - sin(theta_f)) /pi;
 
 %correction factor eta_d
 eta_d = 0.8; %simplified fucntion
 %3D effectiveness value
 k3D = 1.2; %example value
 %calc DeltaCL
 
 DeltaCL = CL_alpha *tau * eta_d * k3D * delta_rad;
 
 DeltaCD = 1.7* (cf/c)^1.38 * (Sf / S_FE) * sin(delta_rad)^2;
 
 %Moment calcs for each fin
 numerator = -2*sin(theta_f) - sin(2*theta_f);
 denominator = 8 * (pi - theta_f + sin(theta_f));
 
 ratio = numerator/denominator;
 
 DeltaCM1_4 = ratio*DeltaCL;
 
 %Deflection angels degrees
 theta = [45, 135, 225, 315];
 
 %initialize force and moment arrays
 
 Fx = zeros(1,4);
 Fy = zeros(1,4);
 Fz = zeros(1,4);
 
 L = zeros(1,4);
 M = zeros(1,4);
 N = zeros(1,4);
 
 %calc forces and moements for each fin
 
 for i = 1:4
     %conv theta to radians
     theta_rad = deg2rad(theta(i));
 
     %calc forces
     Fx(i) = -0.5 * rho * V_bar^2 *Sf*DeltaCD;
     Fy(i) = 0.5*rho*V_bar^2*Sf*(DeltaCL *sin(theta_rad)+ DeltaCD * cos(theta_rad));
     Fz(i) = -0.5 * rho * V_bar^2 *Sf*(DeltaCL *cos(theta_rad)- DeltaCD * sin(theta_rad));
 
     L(i) = Fz(i); %Assume y_i = 1 for simplicity
     M(i) = 0.5*rho*V_bar^2*Sf*c*DeltaCM1_4;
     N(i) = Fy(i); %Assume x_i = 1 for simplicity 
 end
 % Totals
 TotalFx = sum(Fx(:));
 TotalFy = sum(Fy(:));
 TotalFz = sum(Fz(:));

 TotalL = sum(L(:));
 TotalM = sum(M(:));
 TotalN = sum(N(:));
 tau_C = [TotalFx TotalFy TotalFz TotalL TotalM TotalN]';


end
%For natural response 
%tau_C = [0 0 0 0 0 0]';
%}

== matlab function Airship_nonlinear_dynamics_simulink/Airship_model/nonlinear dynamics piecewise3/tau_G ==
  data: rho input; tau_G output size=[6, 1]; m input; g input; VB input; rGx input; g_cap input
function tau_G = fcn(rho, m, g, VB, rGx, g_cap)
%% Gravitational forces and moments
w = m*g;

FG = w*g_cap; % Weight component in body frame (N)
tau_G = [FG; rGx*FG];
end

== matlab function Airship_nonlinear_dynamics_simulink/Airship_model/nonlinear dynamics piecewise3/tau_I ==
  data: J input; tau_I output size=[6, 1]; rGx input; p input; q input; r input; V input; omg input; m input
function tau_I = fcn(J, rGx, p, q, r, V, omg,m)
%% Inertial forces (N) and moments (N-m)
omgx = [0 -omg(3) omg(2) ; omg(3) 0 -omg(1) ; -omg(2) omg(1) 0];

tau_I = [-m*omgx*V + m*omgx*rGx*omg ; -m*rGx*omgx*V - omgx*J*omg];
end

== matlab function Airship_nonlinear_dynamics_simulink/MATLAB Function ==
  data: t input; y output
function y = fcn(t)
if t < 5 
    y = 5; 
elseif t < 15 
    y = 0; 
elseif t < 20
    y = -5; 
elseif t < 30
    y = 0; 
elseif t <35 
    y = -5; 
elseif t <45 
    y = 0; 
elseif t <50 
    y = 5; 
elseif t<60
    y=-0;

else 
    y = 0;
end 
end

== matlab function Airship_nonlinear_dynamics_simulink/Airship_model1/Euler angle estimation5 ==
  data: phi input; EA_dot output; theta input; psi input; p input; q input; r input
function EA_dot = Euler_angle_estimation(phi, theta, psi,p, q, r)


E_dot = [1, sin(phi)* tan(theta) , cos(phi)*tan(theta);
         0, cos(phi) , -sin(phi);
         0, sin(phi)/cos(theta), cos(phi)/cos(theta)];

body_rates = [p; q; r];

EA_dot = transpose(E_dot*body_rates);

end

== matlab function Airship_nonlinear_dynamics_simulink/Airship_model1/Position wrt earth5 ==
  data: u input; XYZ_dot output; v input; w input; phi input; theta input; psi input
function XYZ_dot = position_wrt_Earth(u,v,w,phi,theta,psi)


R_be = [cos(theta)*cos(psi) , sin(theta)*sin(phi)*cos(psi) - cos(theta)*sin(psi), cos(phi)*cos(psi)*sin(theta)+ sin(phi)*sin(psi); ...
    cos(theta)*sin(psi), sin(phi)*sin(theta)*sin(psi) + cos(phi)*cos(psi), cos(phi)*sin(theta)*sin(psi) - sin(phi)*cos(psi); ...
    -sin(theta) , sin(phi)*cos(theta) , cos(phi)*cos(theta)];

body_velocity = [u; v; w];
XYZ_dot = transpose(R_be*body_velocity);
end

== matlab function Airship_nonlinear_dynamics_simulink/Airship_model1/nonlinear dynamics piecewise3/MAH ==
  data: MAH output; g input; L input; D input; k1 input; k2 input; k_dash input; VB input; rho input
function MAH = fcn(g, L, D, k1, k2, k_dash, VB, rho)
%% Estimation of added mass matrix
% MAH - added mass of airship hull
B = VB*rho*g; %Bouyancy force
m_dash = B/g;
%I_dash = sum(m_dash * (L.^2 + D^2) / 20); 
I_dash = (m_dash * (L.^2 + D^2) / 20); 

mH11 = k1*m_dash;
mH22 = k2*m_dash;
mH33 = mH22;
mH44 = 0;
mH55 = k_dash*I_dash;
mH66 = mH55;
mH = [mH11, mH22, mH33, mH44, mH55, mH66];

MAH = diag(mH); %6x6 diagonal matrix
end

== matlab function Airship_nonlinear_dynamics_simulink/Euler angle estimation1 ==
  data: phi input; EA_dot output; theta input; psi input; p input; q input; r input
function EA_dot = Euler_angle_estimation(phi, theta, psi,p, q, r)


E_dot = [1, sin(phi)* tan(theta) , cos(phi)*tan(theta);
         0, cos(phi) , -sin(phi);
         0, sin(phi)/cos(theta), cos(phi)/cos(theta)];

body_rates = [p; q; r];

EA_dot = transpose(E_dot*body_rates);

end

== matlab function Airship_nonlinear_dynamics_simulink/Airship_model1/nonlinear dynamics piecewise3/MATLAB Function10 ==
  data: u input; V output; v input; w input
function V = fcn(u, v, w)
V = [u v w]';
end

== matlab function Airship_nonlinear_dynamics_simulink/Airship_model1/nonlinear dynamics piecewise3/MATLAB Function11 ==
  data: V input; r input; tau_V output size=[6,1]; MVN input; FVN input
 function tau_V = fcn(V, r, MVN, FVN)
 u= V(1); 
 v = V(2);
 w= V(3);

 if v == 0 && w == 0
     FV = [0 0 0]';
     MV = [0 0 0]';
 else
     FV = FVN.*[-u (-v) (-w) ]';
     %FV = FVN*[0 (-v/sqrt(v^2 + w^2)) (-w/sqrt(v^2 +w^2)) ]';
     %MV = MVN*[0 (w/sqrt(v^2 + w^2)) (-v/sqrt(v^2 +w^2)) ]';
    MV = MVN.*[0 (w) (-v) ]'; %make first element function of p if roll oscilations persists

 end
 MV(3) = MV(3) - MVN(3) * r; 
 tau_V = [FV; MV];
 %tau_V = [0 0 0 0 0 0]'; %if slow speed
 
 end

== matlab function Airship_nonlinear_dynamics_simulink/Airship_model1/nonlinear dynamics piecewise3/MATLAB Function14 ==
  data: altitude input; rho output; rho_0 input
function rho = fcn(altitude, rho_0)
    % Constants
    T0 = 288.15;     % K
    L = 0.0065;      % K/m
    g = 9.80665;     % m/s^2
    R = 287.05;      % J/kg.K
%altitude = max(0, altitude);  % keep ≥ 0, but not forcefully clipped
    term = 1 - (L * altitude) / T0;
%rho= rho_0;
    if term <= 0
        rho = 0;
    else
       rho = rho_0 * term^(g / (R * L));
    end
end

== matlab function Airship_nonlinear_dynamics_simulink/Airship_model1/nonlinear dynamics piecewise3/MATLAB Function15 ==
  data: p input; omg output; q input; r input
function omg = fcn(p, q, r)
omg = [p q r]';
end

== matlab function Airship_nonlinear_dynamics_simulink/Airship_model1/nonlinear dynamics piecewise3/MATLAB Function2 ==
  data: rGxm input; rGx output
function rGx = fcn(rGxm)
rGx = [0 -rGxm(3) rGxm(2) ; rGxm(3) 0 -rGxm(1) ; -rGxm(2) rGxm(1) 0];

end

== matlab function Airship_nonlinear_dynamics_simulink/Airship_model1/nonlinear dynamics piecewise3/MATLAB Function3 ==
  data: Ixx input; J output; Iyy input; Izz input; Ixy input; Ixz input; Iyz input
function J = fcn(Ixx, Iyy, Izz, Ixy, Ixz, Iyz)
J = [ Ixx, Ixy, Ixz ; Ixy, Iyy, Iyz ; Ixz, Iyz, Izz];
end

== matlab function Airship_nonlinear_dynamics_simulink/Airship_model1/nonlinear dynamics piecewise3/MATLAB Function4 ==
  data: m input; Mrigid output; I33 input; rGx input; J input
function Mrigid = fcn(m, I33, rGx, J)
Mrigid = [m*I33, -m*rGx; m*rGx,  J];

end

== matlab function Airship_nonlinear_dynamics_simulink/Airship_model1/nonlinear dynamics piecewise3/MATLAB Function6 ==
  data: phi input; g_cap output; theta input
function g_cap = fcn(phi, theta)
    g_cap = [-sin(theta), cos(theta)*sin(phi), cos(theta)*cos(phi)]';
end

== matlab function Airship_nonlinear_dynamics_simulink/Airship_model1/nonlinear dynamics piecewise3/MATLAB Function7 ==
  data: rTDF1 input; tau_Th output; rTDF2 input; fProp1 input; fProp2 input; etaTDF input; Prop1_alpha input; Prop2_alpha input
function tau_Th = fcn(rTDF1, rTDF2, fProp1, fProp2, etaTDF, Prop1_alpha, Prop2_alpha)
%% Airship thrust force and moments


FTDF1 = etaTDF * [fProp1*cos(Prop1_alpha) 0 -fProp1*sin(Prop1_alpha)]'; %Thrust force N
FTDF2 = etaTDF * [fProp2*cos(Prop2_alpha) 0 -fProp2*sin(Prop2_alpha)]';
FTDF = FTDF1+FTDF2;
MTDF1 = cross(rTDF1, FTDF1); %Moments N-m
MTDF2 = cross(rTDF2, FTDF2);
MTDF = MTDF1 + MTDF2;

tau_Th = [FTDF; MTDF];
end

== matlab function Airship_nonlinear_dynamics_simulink/Airship_model1/nonlinear dynamics piecewise3/V_dot out ==
  data: MAH input; V_dot output; MAF input; Mrigid input; tau_I input; tau_G input; tau_C input; tau_AS input; tau_A_dash input; tau_Th input; tau_V input
function V_dot = fcn(MAH, MAF, Mrigid,tau_I, tau_G, tau_C, tau_AS, tau_A_dash, tau_Th, tau_V)
%% Return
V_dot = zeros(6,1);
MA_rigid = (MAH+MAF);
%                                       +tau_Imp for gusts
V_dot = (MA_rigid + Mrigid) \ (tau_I + tau_G + tau_C + tau_AS + tau_A_dash + tau_Th + tau_V);
end

== matlab function Airship_nonlinear_dynamics_simulink/Airship_model1/nonlinear dynamics piecewise3/tau_AS ==
  data: rho input; tau_AS output size=[6, 1]; g input; VB input; g_cap input; rho_he input
function tau_AS = fcn(rho, g, VB, g_cap, rho_he)
%% Aerostatic forces and moments

% first three are forces along x y z
% next three are moments along x y z 
rv = [0 0 0]'; %Since body frame is established at CV, the position ...
FAS = -(rho)*g*VB*g_cap; %Aerostatic forces N
%FAS = -((rho - rho_he) * g * VB) * g_cap;

tau_AS = [FAS; cross(rv,FAS)]; %Aerostatic forces and moments
end

== matlab function Airship_nonlinear_dynamics_simulink/Airship_model1/nonlinear dynamics piecewise3/tau_A_dash ==
  data: MA_rigid input; tau_A_dash output size=[6, 1]; omg input; V input
function tau_A_dash = fcn(MA_rigid, omg, V)
%% Aerodynamic forces and moments
% symmetric added mass axis
% Aerodynamic forces N and moments N-m

% Extract components from the symmetric added mass axis
M11 = MA_rigid(1:3, 1:3);
M12 = MA_rigid(1:3, 4:6);
M21 = MA_rigid(4:6, 1:3);
M22 = MA_rigid(4:6, 4:6);

% Calc aero forces and moments
forces_due_to_rotation = cross(omg, (M11 * V + M12 * omg));
moments_due_to_translation = cross(V, (M11 * V + M12 * omg));
moments_due_to_rotation = cross(omg, (M21 * V + M22 * omg));

% --- Pitch rate damping (natural, from hull and fins) ---
% Set this value using data for your airship (e.g. Skyship-500: -1.2e6 N·m·s/rad)
Mq = -1.2e6; % [N·m·s/rad] (example value, replace with your own if needed)
Mp = -1.2e6; % [N·m·s/rad] (example value, replace with your own if needed)

p = omg(1);

q = omg(2);  % Pitch rate (rad/s)
M_pitch_damping = Mq * q; % Negative sign already in Mq
M_yaw_damping = Mp * p; % Negative sign already in Mq

% Add pitch damping to the moment vector [L; M; N]
moments_due_to_pitch_damping = [0; M_pitch_damping; 0];
moments_due_to_yaw_damping = [M_yaw_damping;0; 0];

% Combine into aero forces and moments (sign change - to +)
tau_A_dash = [forces_due_to_rotation;
              moments_due_to_translation + moments_due_to_rotation + moments_due_to_pitch_damping+moments_due_to_yaw_damping];
end
